simulink model "Bitonic_Sort_Ex1"  (R2025a)
settings: Solver=VariableStepAuto  StartTime=0.0  StopTime=128/100e6  RelTol=1e-3
undefined symbols (not defined in the file): i, nsvg1369, S, xcve1752
libraries: aieDSP x1, commrandsrc3 x1, dspstat3 x1, vmcUtilities x1
settings Model: Creator=sdegala  LastModifiedBy=robg
settings ModelReferenceCC: EnableRefExpFcnMdlSchedulingChecks=on
settings RTWCC: GPUComputeCapability=3.5

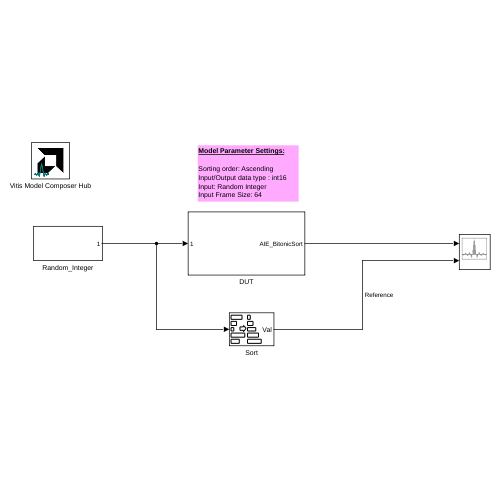
[thumbnail: Simulink's stored preview of the top-level diagram]
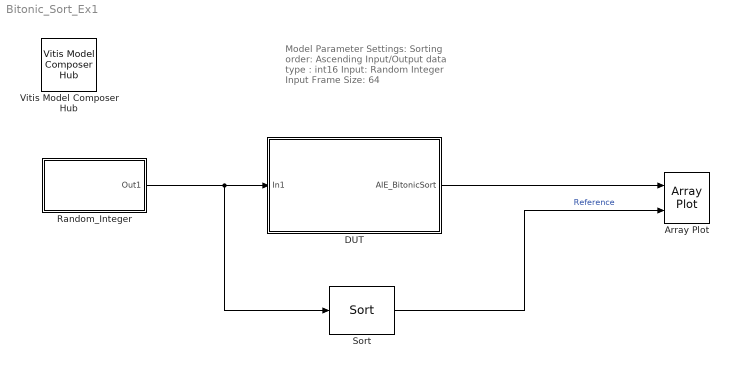
== system Bitonic_Sort_Ex1 ==
  note: Model Parameter Settings:
      |
      | Sorting order: Ascending
      | Input/Output data type : int16
      | Input: Random Integer
      | Input Frame Size: 64
  Array Plot : ArrayPlot  NumInputPorts=2  WindowPosition=[565.000000,321.000000,800.000000,500.000000,]  ScopeFrameLocation=window  YLimits=[-3.875 34.875]  ShowLegend=on
  DUT : Subsystem
  Random_Integer : Subsystem
  Sort : dspstat3/Sort  otype=Value  dir=Ascending  sortAlg=Quick sort  roundingMode=Floor  overflowMode=off  accumDataTypeStr=Inherit: Same as product output  accumLastDataTypeStr=Inherit: Same as product output
  Vitis Model Composer Hub : vmcUtilities/Vitis Model Composer Hub  Tag=genX  CodeGeneration=off  StartColumn=1  NumberOfColumns=1  TargetDirectory=./code  exportDesign=off  analyzeDesign=off  validateDesignOnHw=off  ExportType=AI Engines  IpVendor=xilinx.com  IpLibrary=hls  IpVersion=1.0  IpHWLanguage=Verilog  AieCompilerOptions={}  AieSimulatorOptions={}  CreateTestbench=off  TestbenchStackSize=10  RunRtlSim=off  RunCSim=off  RunAieSim=off  enableSimulationTimeout=on  enableGraphIterations=on  AieSimTimeout=50000  AieGraphIterations=-1  RunAieSimProfiling=off  LaunchVitisAnalyzer=off  PlotOutput=off  RunX86Sim=off  X86SimTimeout=10  GenHwImage=off  GenLibadfXo=off  GenHwValidationCode=off  PlatformType=Not Specified  HwSystemType=Baremetal  HwValidationTarget=hw  ProjDevice=xcve1752-nsvg1369-1MP-i-S  ProjDevicePart=xcve1752-nsvg1369-1MP-i-S  AIEType=AIE  SamplePeriod=-1  ClockFrequency=200  DataPathParallelism=1  xilinxfamily=versalaiedge  part=xcve1752  speed=-1MP-i-S  package=nsvg1369  directory=./netlist  testbench=off  incr_netlist=off  synthesis_tool=Vivado  clock_wrapper=Clock Enables  dbl_ovrd=According to Block Masks  dcm_input_clock_period=10  sysclk_period=10  simulink_period=1  eval_field=0  LogFileName=''  NThreads=4
  wires:
  Sort/1 -> Array Plot/2  "Reference"
  Random_Integer/1(Out1) -> DUT/1(In1), Sort/1
  DUT/1(AIE_BitonicSort) -> Array Plot/1

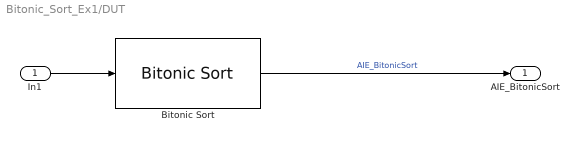
== system Bitonic_Sort_Ex1/DUT ==
  In1 : Inport
  Bitonic Sort : aieDSP/Bitonic Sort  AIE_VARIANT=1  data_type=int16  sample_size=64  num_frames=1  casc_length=1  sort_order=Ascending  ssr=1  blockJsonConstraints=[]  blockJsonConstraintsInternal=[]  spec=vmc_bitonic_sort.json  SerializedMaskParamNames=[]  SerializedMaskParamValues=[]  SerializedMaskParamVisibilities=[]  block_type=Bitonic Sort  SerializedMaskParamDataypes=uint|typename|uint|uint|uint|uint|uint  SerializedMaskParamEnumStrArr=0|0|0|0|0|Descending,Ascending|0  SerializedMaskParamEnumValArr=0|0|0|0|0|0,1|0  SerializedMaskParamVectorArr=0|0|0|0|0|0|0  SerializedMaskParamKeys=AIE_VARIANT|TT_DATA|TP_DIM|TP_NUM_FRAMES|TP_CASC_LEN|TP_ASCENDING|TP_SSR
  AIE_BitonicSort : Outport
  wires:
  In1/1 -> Bitonic Sort/1
  Bitonic Sort/1 -> AIE_BitonicSort/1  "AIE_BitonicSort"

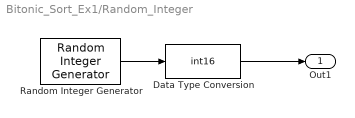
== system Bitonic_Sort_Ex1/Random_Integer ==
  Data Type Conversion : DataTypeConversion  OutDataTypeStr=int16  ConvertRealWorld=Stored Integer (SI)  SaturateOnIntegerOverflow=off  RndMeth=Floor
  Random Integer Generator : commrandsrc3/Random Integer Generator  SetSize=64  SeedSource=Auto  Seed=0  SampleTime=1/100e6  SamplesPerFrame=64  OutputDataType=single  SimulateUsing=Interpreted execution
  Out1 : Outport
  wires:
  Random Integer Generator/1 -> Data Type Conversion/1
  Data Type Conversion/1 -> Out1/1
